simulink model "Quadrocopter_driftsim"  (Simulink 7.4)
settings: Solver=ode45  StartTime=0.0  StopTime=10.0  RelTol=1e-3
values from neighbouring files (symbols this model uses):
  Ts = 0.01    [Reglerauslegung.m]    (also in Test_Reglerauslegung.m)
undefined symbols (not defined in the file or in its folder): boom, f1, f2, f3, f4, f5, g, I_x, I_y, I_z, m
libraries: Copter_Library x5, dspinverses x1
settings Model: Creator=roczit00  LastModifiedBy=roczit00

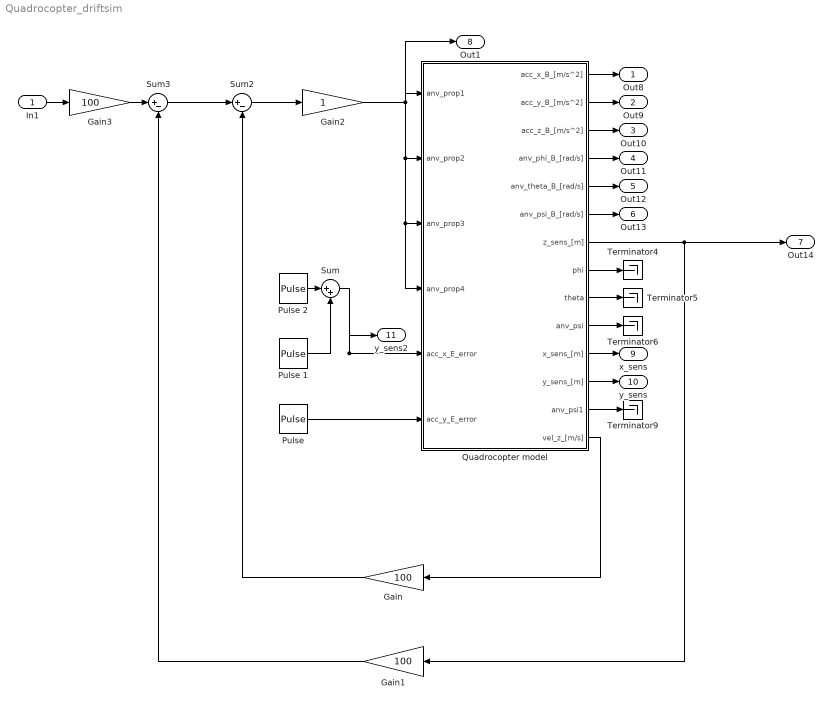
== system Quadrocopter_driftsim ==
  In1 : Inport  OutDataType=fixdt(1, 16)  OutScaling=2^0
  Gain : Gain  Gain=100  ParameterDataType=fixdt(1, 16)  ParameterScaling=2^0  OutDataType=fixdt(1, 16)  OutScaling=2^0
  Gain1 : Gain  Gain=100  ParameterDataType=fixdt(1, 16)  ParameterScaling=2^0  OutDataType=fixdt(1, 16)  OutScaling=2^0
  Gain2 : Gain  ParameterDataType=fixdt(1, 16)  ParameterScaling=2^0  OutDataType=fixdt(1, 16)  OutScaling=2^0
  Gain3 : Gain  Gain=100  ParameterDataType=fixdt(1, 16)  ParameterScaling=2^0  OutDataType=fixdt(1, 16)  OutScaling=2^0
  Pulse : DiscretePulseGenerator  PulseType=Time based  Amplitude=-0.01  Period=1000  PulseWidth=0.01  PhaseDelay=10  SampleTime=1
  Pulse 1 : DiscretePulseGenerator  PulseType=Time based  Amplitude=0.01  Period=2  PulseWidth=0.01  PhaseDelay=1  SampleTime=1
  Pulse 2 : DiscretePulseGenerator  PulseType=Time based  Amplitude=0.03  Period=1000  PulseWidth=0.01  PhaseDelay=12  SampleTime=1
  Quadrocopter model : Subsystem  AncestorBlock=Copter_Library/Quadrocopter model
  Sum : Sum  Inputs=|++  OutDataType=fixdt(1, 16)  OutScaling=2^0
  Sum2 : Sum  Inputs=|+-  OutDataType=fixdt(1, 16)  OutScaling=2^0
  Sum3 : Sum  Inputs=|+-  OutDataType=fixdt(1, 16)  OutScaling=2^0
  Terminator{4..6,9} (4 alike) : Terminator
  Out8 : Outport  OutDataType=fixdt(1, 16)  OutScaling=2^0
  Out9 : Outport  Port=2  OutDataType=fixdt(1, 16)  OutScaling=2^0
  Out10 : Outport  Port=3  OutDataType=fixdt(1, 16)  OutScaling=2^0
  Out11 : Outport  Port=4  OutDataType=fixdt(1, 16)  OutScaling=2^0
  Out12 : Outport  Port=5  OutDataType=fixdt(1, 16)  OutScaling=2^0
  Out13 : Outport  Port=6  OutDataType=fixdt(1, 16)  OutScaling=2^0
  Out14 : Outport  Port=7  OutDataType=fixdt(1, 16)  OutScaling=2^0
  Out1 : Outport  Port=8  OutDataType=fixdt(1, 16)  OutScaling=2^0
  x_sens : Outport  Port=9  OutDataType=fixdt(1, 16)  OutScaling=2^0
  y_sens : Outport  Port=10  OutDataType=fixdt(1, 16)  OutScaling=2^0
  y_sens2 : Outport  Port=11  OutDataType=fixdt(1, 16)  OutScaling=2^0
  wires:
  Quadrocopter model/8(phi) -> Terminator4/1
  Quadrocopter model/9(theta) -> Terminator5/1
  Quadrocopter model/10(anv_psi) -> Terminator6/1
  Quadrocopter model/1(acc_x_B_[m/s^2]) -> Out8/1
  Quadrocopter model/2(acc_y_B_[m/s^2]) -> Out9/1
  Quadrocopter model/3(acc_z_B_[m/s^2]) -> Out10/1
  Quadrocopter model/4(anv_phi_B_[rad/s]) -> Out11/1
  Quadrocopter model/5(anv_theta_B_[rad/s]) -> Out12/1
  Quadrocopter model/6(anv_psi_B_[rad/s]) -> Out13/1
  Quadrocopter model/11(x_sens_[m]) -> x_sens/1
  Quadrocopter model/12(y_sens_[m]) -> y_sens/1
  Quadrocopter model/13(anv_psi1) -> Terminator9/1
  Quadrocopter model/7(z_sens_[m]) -> Out14/1, Gain1/1
  Quadrocopter model/14(vel_z_[m/s]) -> Gain/1
  Gain1/1 -> Sum3/2
  Gain/1 -> Sum2/2
  Sum3/1 -> Sum2/1
  Sum2/1 -> Gain2/1
  Gain2/1 -> Out1/1, Quadrocopter model/1(anv_prop1), Quadrocopter model/2(anv_prop2), Quadrocopter model/3(anv_prop3), Quadrocopter model/4(anv_prop4)
  In1/1 -> Gain3/1
  Gain3/1 -> Sum3/1
  Pulse/1 -> Quadrocopter model/6(acc_y_E_error)
  Pulse 1/1 -> Sum/2
  Sum/1 -> y_sens2/1, Quadrocopter model/5(acc_x_E_error)
  Pulse 2/1 -> Sum/1

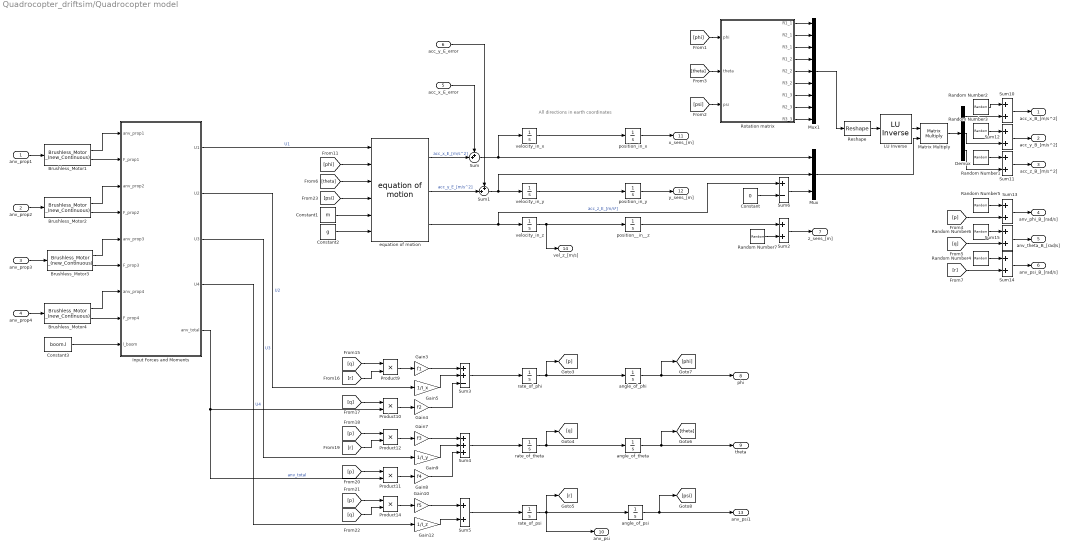
== system Quadrocopter_driftsim/Quadrocopter model ==
  note: All directions in earth coordinates
  anv_prop1 : Inport  OutDataType=fixdt(1, 16)  OutScaling=2^0
  anv_prop2 : Inport  Port=2  OutDataType=fixdt(1, 16)  OutScaling=2^0
  anv_prop3 : Inport  Port=3  OutDataType=fixdt(1, 16)  OutScaling=2^0
  anv_prop4 : Inport  Port=4  OutDataType=fixdt(1, 16)  OutScaling=2^0
  acc_x_E_error : Inport  Port=5  OutDataType=fixdt(1, 16)  OutScaling=2^0
  acc_y_E_error : Inport  Port=6  OutDataType=fixdt(1, 16)  OutScaling=2^0
  " LU Inverse" : dspinverses/ LU Inverse  SystemSampleTime=-1
  Brushless_Motor{1..4} (4 alike) : Copter_Library/Brushless_Motor _(new_Continuous)  SystemSampleTime=-1
  Constant : Constant  Value=0  OutDataType=fixdt(1, 16)  OutScaling=2^0  SampleTime=Ts
  Constant1 : Constant  Value=m  OutDataType=fixdt(1, 16)  OutScaling=2^0  SampleTime=Ts
  Constant2 : Constant  Value=g  OutDataType=fixdt(1, 16)  OutScaling=2^0  SampleTime=Ts
  Constant3 : Constant  Value=boom.l  OutDataType=fixdt(1, 16)  OutScaling=2^0
  Demux : Demux  Outputs=3
  Gain10 : Gain  Gain=f5  ParameterDataType=fixdt(1, 16)  ParameterScaling=2^0  OutDataType=fixdt(1, 16)  OutScaling=2^0
  Gain12 : Gain  Gain=1/I_z  ParameterDataType=fixdt(1, 16)  ParameterScaling=2^0  OutDataType=fixdt(1, 16)  OutScaling=2^0
  Gain3 : Gain  Gain=f1  ParameterDataType=fixdt(1, 16)  ParameterScaling=2^0  OutDataType=fixdt(1, 16)  OutScaling=2^0
  Gain4 : Gain  Gain=f2  ParameterDataType=fixdt(1, 16)  ParameterScaling=2^0  OutDataType=fixdt(1, 16)  OutScaling=2^0
  Gain5 : Gain  Gain=1/I_x  ParameterDataType=fixdt(1, 16)  ParameterScaling=2^0  OutDataType=fixdt(1, 16)  OutScaling=2^0
  Gain7 : Gain  Gain=f3  ParameterDataType=fixdt(1, 16)  ParameterScaling=2^0  OutDataType=fixdt(1, 16)  OutScaling=2^0
  Gain8 : Gain  Gain=f4  ParameterDataType=fixdt(1, 16)  ParameterScaling=2^0  OutDataType=fixdt(1, 16)  OutScaling=2^0
  Gain9 : Gain  Gain=1/I_y  ParameterDataType=fixdt(1, 16)  ParameterScaling=2^0  OutDataType=fixdt(1, 16)  OutScaling=2^0
  Input Forces and Moments : Stateflow chart
  Matrix Multiply : Product  Multiplication=Matrix(*)  OutDataType=sfix(16)  OutScaling=2^0
  Mux : Mux  Inputs=3
  Mux1 : Mux  Inputs=9
  Product{9..12,14} (5 alike) : Product  OutDataType=fixdt(1, 16)  OutScaling=2^0  RndMeth=Zero
  Random Number1 : RandomNumber  Variance=0.0018105  Seed=4684684654  SampleTime=Ts
  Random Number2 : RandomNumber  Variance=0.0003  Seed=456456465  SampleTime=0.01
  Random Number3 : RandomNumber  Variance=0.0003  Seed=676764  SampleTime=Ts
  Random Number{4..7} (4 alike) : RandomNumber  Variance=0  SampleTime=Ts
  Reshape : Reshape  OutputDimensionality=Customize  OutputDimensions=[3,3]
  Rotation matrix : Stateflow chart
  Sum : Sum  Inputs=++|  OutDataType=fixdt(1, 16)  OutScaling=2^0
  Sum1 : Sum  Inputs=++|  OutDataType=fixdt(1, 16)  OutScaling=2^0
  Sum{2,5,10..15} (8 alike) : Sum  OutDataType=fixdt(1, 16)  OutScaling=2^0
  Sum3 : Sum  Inputs=++-  OutDataType=fixdt(1, 16)  OutScaling=2^0
  Sum4 : Sum  Inputs=+++  OutDataType=fixdt(1, 16)  OutScaling=2^0
  Sum6 : Sum  Inputs=+-  OutDataType=fixdt(1, 16)  OutScaling=2^0
  angle_of_phi : Integrator
  angle_of_psi : Integrator
  angle_of_theta : Integrator
  equation of motion : Copter_Library/equation of motion  SystemSampleTime=-1
  position__in__z : Integrator
  position_in_x : Integrator
  position_in_y : Integrator
  rate_of_phi : Integrator
  rate_of_psi : Integrator
  rate_of_theta : Integrator
  velocity_in_x : Integrator
  velocity_in_y : Integrator
  velocity_in_z : Integrator
  acc_x_B_[m/s^2] : Outport  OutDataType=fixdt(1, 16)  OutScaling=2^0
  acc_y_B_[m/s^2] : Outport  Port=2  OutDataType=fixdt(1, 16)  OutScaling=2^0
  acc_z_B_[m/s^2] : Outport  Port=3  OutDataType=fixdt(1, 16)  OutScaling=2^0
  anv_phi_B_[rad/s] : Outport  Port=4  OutDataType=fixdt(1, 16)  OutScaling=2^0
  anv_theta_B_[rad/s] : Outport  Port=5  OutDataType=fixdt(1, 16)  OutScaling=2^0
  anv_psi_B_[rad/s] : Outport  Port=6  OutDataType=fixdt(1, 16)  OutScaling=2^0
  z_sens_[m] : Outport  Port=7  OutDataType=fixdt(1, 16)  OutScaling=2^0
  phi : Outport  Port=8  OutDataType=fixdt(1, 16)  OutScaling=2^0
  theta : Outport  Port=9  OutDataType=fixdt(1, 16)  OutScaling=2^0
  anv_psi : Outport  Port=10  OutDataType=fixdt(1, 16)  OutScaling=2^0
  x_sens_[m] : Outport  Port=11  OutDataType=fixdt(1, 16)  OutScaling=2^0
  y_sens_[m] : Outport  Port=12  OutDataType=fixdt(1, 16)  OutScaling=2^0
  anv_psi1 : Outport  Port=13  OutDataType=fixdt(1, 16)  OutScaling=2^0
  vel_z_[m/s] : Outport  Port=14  OutDataType=fixdt(1, 16)  OutScaling=2^0
  wires:
  Random Number7/1 -> Sum2/2
  Sum2/1 -> z_sens_[m]/1
  position__in__z/1 -> Sum2/1
  acc_y_E_error/1 -> Sum1/1
  acc_x_E_error/1 -> Sum/1
  Sum/1 -> velocity_in_x/1, Mux/1
  equation of motion/1 -> Sum/2  "acc_x_E_[m/s^2]"
  equation of motion/2 -> Sum1/2  "acc_y_E_[m/s^2]"
  Sum1/1 -> Mux/2, velocity_in_y/1
  position_in_y/1 -> y_sens_[m]/1
  position_in_x/1 -> x_sens_[m]/1
  equation of motion/3 -> Sum6/1, velocity_in_z/1  "acc_z_E_[m/s²]"
  Constant2/1 -> equation of motion/6
  Constant1/1 -> equation of motion/5
  [psi] -> equation of motion/4
  [theta] -> equation of motion/3
  [phi] -> equation of motion/2
  Brushless_Motor4/2 -> Input Forces and Moments/8(F_prop4)
  Brushless_Motor4/1 -> Input Forces and Moments/7(anv_prop4)
  Brushless_Motor3/2 -> Input Forces and Moments/6(F_prop3)
  Brushless_Motor3/1 -> Input Forces and Moments/5(anv_prop3)
  Brushless_Motor2/2 -> Input Forces and Moments/4(F_prop2)
  Brushless_Motor2/1 -> Input Forces and Moments/3(anv_prop2)
  Brushless_Motor1/2 -> Input Forces and Moments/2(F_prop1)
  Brushless_Motor1/1 -> Input Forces and Moments/1(anv_prop1)
  " LU Inverse"/1 -> Matrix Multiply/1
  Sum6/1 -> Mux/3
  Constant/1 -> Sum6/2
  rate_of_psi/1 -> [r], angle_of_psi/1, anv_psi/1
  rate_of_theta/1 -> [q], angle_of_theta/1
  rate_of_phi/1 -> angle_of_phi/1, [p]
  angle_of_psi/1 -> [psi], anv_psi1/1
  angle_of_theta/1 -> theta/1, [theta]
  angle_of_phi/1 -> phi/1, [phi]
  Input Forces and Moments/5(anv_total) -> Product10/2, Product11/2  "anv_total"
  [q] -> Product9/1
  [r] -> Product9/2
  Product9/1 -> Gain3/1
  Gain3/1 -> Sum3/1
  [q] -> Product10/1
  Product10/1 -> Gain4/1
  Input Forces and Moments/2(U2) -> Gain5/1  "U2"
  Gain5/1 -> Sum3/2
  Gain4/1 -> Sum3/3
  Sum3/1 -> rate_of_phi/1
  Input Forces and Moments/1(U1) -> equation of motion/1  "U1"
  [p] -> Product12/1
  [r] -> Product12/2
  Product12/1 -> Gain7/1
  Gain7/1 -> Sum4/1
  [p] -> Product11/1
  Product11/1 -> Gain8/1
  Gain9/1 -> Sum4/2
  Gain8/1 -> Sum4/3
  Input Forces and Moments/3(U3) -> Gain9/1  "U3"
  Sum4/1 -> rate_of_theta/1
  [p] -> Product14/1
  [q] -> Product14/2
  Product14/1 -> Gain10/1
  Gain10/1 -> Sum5/1
  Gain12/1 -> Sum5/2
  Input Forces and Moments/4(U4) -> Gain12/1  "U4"
  Sum5/1 -> rate_of_psi/1
  Constant3/1 -> Input Forces and Moments/9(l_boom)
  velocity_in_z/1 -> position__in__z/1, vel_z_[m/s]/1
  velocity_in_y/1 -> position_in_y/1
  velocity_in_x/1 -> position_in_x/1
  anv_prop1/1 -> Brushless_Motor1/1
  anv_prop2/1 -> Brushless_Motor2/1
  [phi] -> Rotation matrix/1(phi)
  [theta] -> Rotation matrix/2(theta)
  [psi] -> Rotation matrix/3(psi)
  Rotation matrix/1(R1_1) -> Mux1/1
  Rotation matrix/2(R2_1) -> Mux1/2
  Rotation matrix/3(R3_1) -> Mux1/3
  Rotation matrix/4(R1_2) -> Mux1/4
  Rotation matrix/5(R2_2) -> Mux1/5
  Rotation matrix/6(R3_2) -> Mux1/6
  Rotation matrix/7(R1_3) -> Mux1/7
  Rotation matrix/8(R2_3) -> Mux1/8
  Rotation matrix/9(R3_3) -> Mux1/9
  Mux1/1 -> Reshape/1
  Mux/1 -> Matrix Multiply/2
  Reshape/1 -> " LU Inverse"/1
  anv_prop4/1 -> Brushless_Motor4/1
  anv_prop3/1 -> Brushless_Motor3/1
  Matrix Multiply/1 -> Demux/1
  Random Number2/1 -> Sum10/1
  Demux/1 -> Sum10/2
  Random Number1/1 -> Sum11/1
  Demux/3 -> Sum11/2
  Random Number3/1 -> Sum12/1
  Demux/2 -> Sum12/2
  Sum10/1 -> acc_x_B_[m/s^2]/1
  Sum12/1 -> acc_y_B_[m/s^2]/1
  Sum11/1 -> acc_z_B_[m/s^2]/1
  Random Number5/1 -> Sum13/1
  [p] -> Sum13/2
  Random Number4/1 -> Sum14/1
  [r] -> Sum14/2
  Random Number6/1 -> Sum15/1
  [q] -> Sum15/2
  Sum13/1 -> anv_phi_B_[rad/s]/1
  Sum15/1 -> anv_theta_B_[rad/s]/1
  Sum14/1 -> anv_psi_B_[rad/s]/1

== matlab function Quadrocopter model/Input Forces and Moments ==
  data: anv_prop1 input double; F_prop1 input double; anv_prop2 input double; F_prop2 input double; anv_prop3 input double; F_prop3 input double; anv_prop4 input double; U1 output double; F_prop4 input double; U2 output double; U3 output double; U4 output double; l_boom input double; anv_total output double
function [U1, U2, U3, U4, anv_total] = input(anv_prop1,F_prop1,anv_prop2,...
    F_prop2,anv_prop3,F_prop3,anv_prop4,F_prop4,l_boom)
%#eml

% Calculating Thrust in z-axis with respect to body fixed coordinate system
U1 = F_prop1 + F_prop2 + F_prop3 + F_prop4;             % [N]

% Calculating Torque around x-axis (Roll) due to Thrust
U2 = l_boom*(-F_prop4+F_prop2);                         % [Nm]

% Calculating Torque around y-axis (Pitch) due to Thrust
U3 = l_boom*(-F_prop1+F_prop3);                         % [Nm]

% Calculating Torque around z-axis (Yaw) due to Thrust
U4 = l_boom*(F_prop1-F_prop2+F_prop3-F_prop4);          % [Nm]

% Overall propeller speed
anv_total = anv_prop1-anv_prop2+anv_prop3-anv_prop4;    % [rad/s]

== matlab function Quadrocopter model/Rotation matrix ==
  data: phi input double; theta input double; psi input double; R1_1 output double; R2_1 output double; R3_1 output double; R1_2 output double; R2_2 output double; R3_2 output double; R1_3 output double; R2_3 output double; R3_3 output double
function [ R1_1, R2_1, R3_1, R1_2, R2_2, R3_2, R1_3, R2_3, R3_3] = input...
                                                    (phi, theta, psi)
% Transformation of E-frame to B-Frame
R1_1 = cos(psi)*cos(theta);
R2_1 = sin(psi)*cos(theta);
R3_1 = -sin(theta);
R1_2 = -sin(psi)*cos(phi)+cos(psi)*sin(theta)*sin(phi);
R2_2 = cos(psi)*cos(phi)+sin(psi)*sin(theta)*sin(phi);
R3_2 = cos(theta)*sin(phi);
R1_3 = sin(psi)*sin(phi)+cos(psi)*sin(theta)*cos(phi);
R2_3 = -cos(psi)*sin(phi)+sin(psi)*sin(theta)*cos(phi);
R3_3 = cos(theta)*cos(phi);
